simulink model "slexMonostaticRadarMultipleTargetsExample"  (R2024b)
settings: Solver=FixedStepDiscrete  StartTime=0.0  StopTime=99/paramRadarMT.prf  RelTol=1e-3  EnableMultiTasking=on
PreLoadFcn:
  | helperslexMonostaticRadarMultipleTargetsParam()
undefined symbols (not defined in the file or in its folder): paramRadarMT, phased
libraries: phasedenvlib x4, phasedtxrxlib x4, phaseddetectlib x3, simulink x1, phasedbflib x1, phasedwavlib x1
CloseFcn:
  | clear paramRadarMT
Description:
  | Monostatic Radar with Three Targets
settings Model: Creator=The MathWorks, Inc.  LastModifiedBy=The MathWorks, Inc.
settings SolverCC: AlgebraicLoopSolver=TrustRegion
settings DataIOCC: LimitDataPoints=on  SaveFormat=Array  SaveOutput=off  SaveTime=off  ReturnWorkspaceOutputs=off
settings OptimizationCC: ExpressionDepthLimit=2147483647  LifeSpan=inf
settings DebuggingCC: ReadBeforeWriteMsg=DisableAll  WriteAfterWriteMsg=DisableAll  WriteAfterReadMsg=DisableAll  UnderspecifiedInitializationDetection=Classic  MergeDetectMultiDrivingBlocksExec=none  SolverPrmCheckMsg=warning  InheritedTsInSrcMsg=none  MultiTaskDSMMsg=none  FcnCallInpInsideContextMsg=warning  UnconnectedInputMsg=warning  UnconnectedOutputMsg=warning  UnconnectedLineMsg=warning  AllowSymbolicDim=off  StateNameClashWarn=warning  SFUnexpectedBacktrackingDiag=warning  SFNoUnconditionalDefaultTransitionDiag=warning  SFExecutionAtInitializationDiag=none  ArithmeticOperatorsInVariantConditions=warning
settings HardwareCC: ProdBitPerPointer=32  ProdBitPerSizeT=32  ProdBitPerPtrDiffT=32  ProdLargestAtomicFloat=None  ProdIntDivRoundTo=Undefined  ProdEndianess=Unspecified  ProdWordSize=32  ProdHWDeviceType=32-bit Generic
settings ModelReferenceCC: UpdateModelReferenceTargets=IfOutOfDate  EnableRefExpFcnMdlSchedulingChecks=on  PropagateSignalLabelsOutOfModel=off
settings SFSimCC: SFSimEcho=off  SimUseLocalCustomCode=off  SimParseCustomCode=off  CustomCodeUndefinedFunction=UseInterfaceOnly
settings RTWCC: RTWUseLocalCustomCode=off  GPUComputeCapability=3.5  DLArmComputeVersion=19.05
settings CodeAppCC: StateflowObjectComments=on
settings GRTTargetCC: TargetLangStandard=C89/C90 (ANSI)  CombineOutputUpdateFcns=off  GRTInterface=on
settings ConfigComp: CovMetricSettings=dw  CovSaveCumulativeToWorkspaceVar=on  CovSaveSingleToWorkspaceVar=on  CovExternalEMLEnable=off  CovSFcnEnable=off

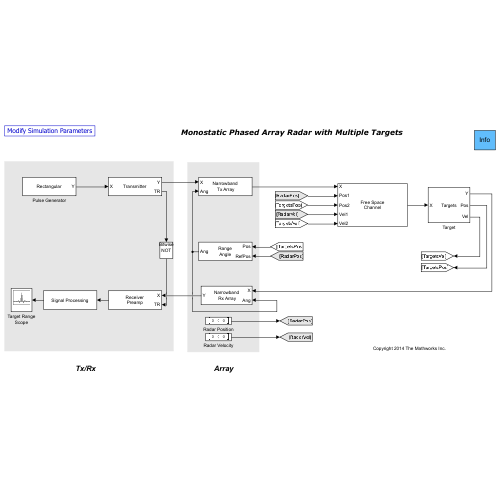
[thumbnail: Simulink's stored preview of the top-level diagram]
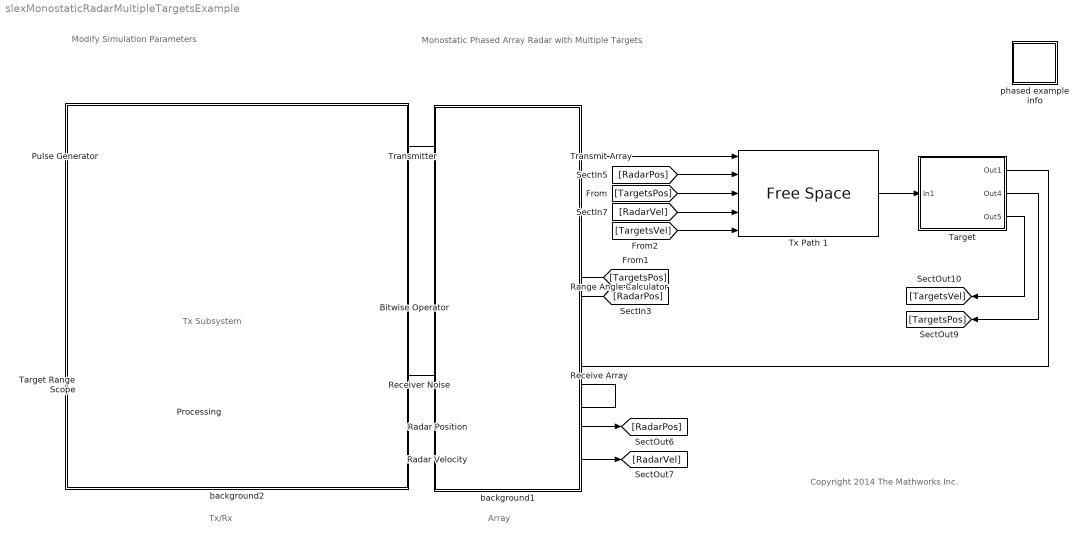
== system slexMonostaticRadarMultipleTargetsExample ==
  note: Monostatic Phased Array Radar with Multiple Targets
  note: Tx Subsystem
  note: Tx/Rx
  note: Modify Simulation Parameters
  note: Copyright 2014 The Mathworks Inc.
  note: Array
  Bitwise Operator : simulink/Logic and Bit Operations/Bitwise Operator  logicop=NOT  UseBitMask=off  BitMask=bin2dec('11011001')  BitMaskRealWorld=Stored Integer
  Processing : Subsystem
      mask Display: disp('Signal Processing')
  Pulse Generator : phasedwavlib/Rectangular Waveform  SampleRate=paramRadarMT.fs  DurationSpecification=Pulse width  PulseWidth=1/paramRadarMT.pulseBw  DutyCycle=0.5  PRF=paramRadarMT.prf  PRFSelectionInputPort=off  SimulationTimeSource=Derive from waveform parameters  FrequencyOffsetSource=Property  FrequencyOffset=0  OutputFormat=Pulses  NumSamples=100  NumPulses=1  PRFOutputPort=off  CoefficientsOutputPort=off  SimulateUsing=Interpreted execution
  Radar Position : Constant  Value=[ 0; 0; 0 ]  SampleTime=1/paramRadarMT.prf
  Radar Velocity : Constant  Value=[ 0; 0; 0 ]  SampleTime=1/paramRadarMT.prf
  Range Angle Calculator : phasedenvlib/Range Angle Calculator  Model=Free space  ReferencePositionSource=Input port  ReferencePosition=[ 0; 0; 0 ]  ReferenceAxesSource=Property  ReferenceAxes=eye( 3 )  Output=Angle  SimulateUsing=Interpreted execution
  Receive Array : phasedtxrxlib/Narrowband Receive Array  PropagationSpeed=paramRadarMT.propSpeed  OperatingFrequency=paramRadarMT.fc  Wavefront=Plane  SensorGainMeasure=dB  Polarization=None  WeightsInputPort=off  SimulateUsing=Interpreted execution  Sensor=phased.ULA('NumElements',4,'Element',phased.IsotropicAntennaElement(),'ElementSpacing',paramRadarMT.lambda/2)
  Receiver Noise : phasedtxrxlib/Receiver Preamp  Gain=20  LossFactor=0  NoiseMethod=Noise temperature  NoiseFigure=0  ReferenceTemperature=290  SampleRateFromInputCheckbox=on  SampleRate=1e6  NoisePower=0  EnableInputPort=on  PhaseNoiseInputPort=off  SeedSource=Auto  Seed=0  SimulateUsing=Interpreted execution
  Target : Subsystem
      mask Display:
      | disp('Targets')
      | port_label('input',1,'X');
      | port_label('output',1,'Y');
      | port_label('output',2,'Pos');
      | port_label('output',3,'Vel');
  Target Range Scope : ArrayPlot  WindowPosition=[838.000000,339.000000,808.000000,454.000000,]  SampleIncrement=paramRadarMT.metersPerSample  XOffset=paramRadarMT.rangeOffset  PlotType=Line  AxesScaling=Manual  Title=Radar Return  XLabel=Range (m)  YLimits=[-4.2427e-08,1.7395e-06]
  Transmit Array : phasedtxrxlib/Narrowband Transmit Array  PropagationSpeed=paramRadarMT.propSpeed  OperatingFrequency=paramRadarMT.fc  CombineRadiatedSignals=on  SensorGainMeasure=dB  Polarization=None  WeightsInputPort=off  SimulateUsing=Interpreted execution  Sensor=phased.ULA('NumElements',4,'Element',phased.IsotropicAntennaElement(),'ElementSpacing',paramRadarMT.lambda/2)
  Transmitter : phasedtxrxlib/Transmitter  PeakPower=paramRadarMT.peakPower/16  GainMethod=Linear  Gain=paramRadarMT.txGain  LossFactor=0  OIP3=Inf  Table=[ -25, 5, -1; -10, 20, -2; 0, 27, 12; 5, 28, 12 ]  InUseOutputPort=on  CoherentOnTransmit=on  PhaseNoiseOutputPort=off  SimulateUsing=Interpreted execution  NoiseMethod=None  NoiseFigure=3  NoiseFactor=2  NoiseTemperature=290  ReferenceTemperature=290  SampleRate=1e6  SampleRateFromInputCheckbox=on  PhaseOffset=0  SeedSource=Auto  Seed=0
  Tx Path 1 : phasedenvlib/Free Space  PropagationSpeed=paramRadarMT.propSpeed  OperatingFrequency=paramRadarMT.fc  TwoWayPropagation=on  SampleRateFromInputCheckbox=on  SampleRate=1e6  MaximumDistanceSource=Property  MaximumDistance=10e3  MaximumNumInputSamplesSource=Auto  MaximumNumInputSamples=1000  SimulateUsing=Interpreted execution
  background1 : Subsystem  Description=Jammer
      mask Display: disp('')
  background2 : Subsystem  Description=Jammer
      mask Display: disp('')
  phased example info : Subsystem
      settings: OpenFcn=|
      | modelname = 'slexMonostaticRadarExample';
      | helpview(fullfile(matlabroot,'help','phased','helptargets.map'),sprintf('%sExample',modelname));
      | clear modelname;
      mask Display: disp('Info')
  wires:
  Pulse Generator/1 -> Transmitter/1
  Receiver Noise/1 -> Processing/1(In1)
  Processing/1(Out1) -> Target Range Scope/1
  Transmitter/1 -> Transmit Array/1
  Receive Array/1 -> Receiver Noise/1
  Bitwise Operator/1 -> Receiver Noise/2
  Range Angle Calculator/1 -> Receive Array/2, Transmit Array/2
  [RadarPos] -> Range Angle Calculator/2
  Transmit Array/1 -> Tx Path 1/1
  [RadarVel] -> Tx Path 1/4
  [TargetsPos] -> Range Angle Calculator/1
  [TargetsVel] -> Tx Path 1/5
  [RadarPos] -> Tx Path 1/2
  Radar Velocity/1 -> [RadarVel]
  Radar Position/1 -> [RadarPos]
  Transmitter/2 -> Bitwise Operator/1
  [TargetsPos] -> Tx Path 1/3
  Tx Path 1/1 -> Target/1(In1)
  Target/2(Out4) -> [TargetsPos]
  Target/3(Out5) -> [TargetsVel]
  Target/1(Out1) -> Receive Array/1

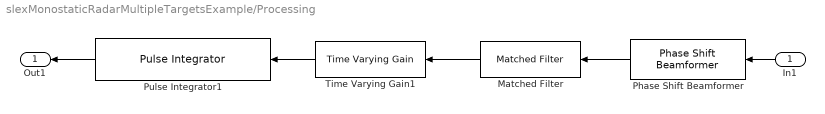
== system slexMonostaticRadarMultipleTargetsExample/Processing ==
  In1 : Inport
  Matched Filter : phaseddetectlib/Matched Filter  CoefficientsSource=Property  Coefficients=paramRadarMT.matchingCoeff  SpectrumWindow=None  CustomSpectrumWindow=@hamming  SpectrumRange=[ 0, 1e5 ]  SampleRateFromInputCheckbox=on  SampleRate=1e6  SidelobeAttenuation=30  Beta=0.5  Nbar=4  GainOutputPort=off  MaximumNumInputSamplesSource=Auto  MaximumNumInputSamples=100  SimulateUsing=Interpreted execution
  Phase Shift Beamformer : phasedbflib/Phase Shift Beamformer  PropagationSpeed=paramRadarMT.propSpeed  OperatingFrequency=paramRadarMT.fc  DirectionSource=Property  Direction=[ 0; 0 ]  NumPhaseShifterBits=0  WeightsNormalization=Distortionless  WeightsOutputPort=off  SimulateUsing=Interpreted execution  SensorArray=phased.ULA('Element',phased.IsotropicAntennaElement(),'NumElements',4,'Taper',1,'ElementSpacing',paramRadarMT.lambda/2)
  Pulse Integrator1 : phaseddetectlib/Pulse Integrator  CoherentFlag=Noncoherent  N=10  V=0
  Time Varying Gain1 : phaseddetectlib/Time Varying Gain  RangeLossSource=Property  RangeLoss=paramRadarMT.rangeLoss  ReferenceLoss=paramRadarMT.referenceLoss  SimulateUsing=Interpreted execution
  Out1 : Outport  VectorParamsAs1DForOutWhenUnconnected=off
  wires:
  Time Varying Gain1/1 -> Pulse Integrator1/1
  Matched Filter/1 -> Time Varying Gain1/1
  Pulse Integrator1/1 -> Out1/1
  In1/1 -> Phase Shift Beamformer/1
  Phase Shift Beamformer/1 -> Matched Filter/1

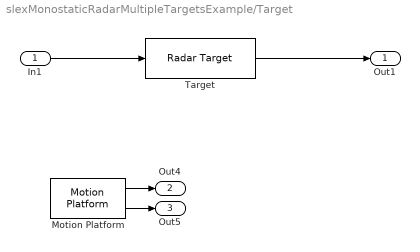
== system slexMonostaticRadarMultipleTargetsExample/Target ==
  In1 : Inport
  Motion Platform : phasedenvlib/Motion Platform  MotionModel=Velocity  InitialPosition=paramRadarMT.targetPos  InitialVelocity=[ 0; 0; 0 ]  VelocitySource=Property  Velocity=paramRadarMT.targetVel  AccelerationSource=Property  Acceleration=[0;0;0]  CustomTrajectory=[ 0, 0, 0, 0, 0, 0, 0; 1, 0, 0, 0, 0, 0, 0 ]  ScanMode=None  InitialScanAngle=0  AzimuthSpan=[ -60, 60 ]  AzimuthScanRate=10  InitialOrientationAxes=eye(3)  OrientationAxesOutputPort=off  ElapsedTimeSource=Auto  SampleRateFromInputCheckbox=on  SampleRate=1e6  SimulateUsing=Interpreted execution
  Target : phasedenvlib/Radar Target  EnablePolarization=off  Mode=Monostatic  MeanRCSSource=Property  ScatteringMatrixSource=Property  MeanRCS=paramRadarMT.targetRcs  ScatteringMatrix=eye( 2 )  Model=Nonfluctuating  PropagationSpeed=paramRadarMT.propSpeed  OperatingFrequency=paramRadarMT.fc  SeedSource=Auto  Seed=0  SimulateUsing=Interpreted execution
  Out1 : Outport  VectorParamsAs1DForOutWhenUnconnected=off
  Out4 : Outport  Port=2  VectorParamsAs1DForOutWhenUnconnected=off
  Out5 : Outport  Port=3  VectorParamsAs1DForOutWhenUnconnected=off
  wires:
  In1/1 -> Target/1
  Target/1 -> Out1/1
  Motion Platform/1 -> Out4/1
  Motion Platform/2 -> Out5/1

== system slexMonostaticRadarMultipleTargetsExample/background1 ==

== system slexMonostaticRadarMultipleTargetsExample/background2 ==

== system slexMonostaticRadarMultipleTargetsExample/phased example info ==
